simulink model "Battery_Model_1cell_param_"  (R2021b)
settings: Solver=ode3  StartTime=0  StopTime=60000  FixedStep=10  RelTol=1e-3
undefined symbols (not defined in the file or in its folder): Cap, Cell_dev_mean, Cell_dev_sigma, Current_exp_high, n_cells, OCV1, OCV10, OCV2, OCV3, OCV4, OCV5, OCV6, OCV7, OCV8, OCV9, pCl1_High, pCl1_Low, pCl1_Mid, pCl2_High, pCl2_Low, pCl2_Mid, pCl3_High, pCl3_Low, pCl3_Mid, pCs1_High, pCs1_Low, pCs1_Mid, pCs2_High, pCs2_Low, pCs2_Mid, pCs3_High, pCs3_Low, pCs3_Mid, pRl1_High, pRl1_Low, pRl1_Mid, pRl2_High, pRl2_Low, pRl2_Mid, pRl3_High, pRl3_Low, pRl3_Mid, pRs1_High, pRs1_Low, pRs1_Mid, pRs2_High, pRs2_Low, pRs2_Mid, pRs3_High, pRs3_Low, pRs3_Mid, pRse1_High, pRse1_Low, pRse1_Mid, pRse2_High, pRse2_Low, pRse2_Mid, pRse3_High, pRse3_Low, pRse3_Mid ... (+6)
libraries: simulink x2, matrix_library x1
(part 1 of 2)
settings Model: Creator=CWI  LastModifiedBy=osy04
settings SolverCC: AlgebraicLoopSolver=TrustRegion
settings DataIOCC: LimitDataPoints=on  SaveFormat=Array  ReturnWorkspaceOutputs=off
settings OptimizationCC: BlockReduction=off  BooleanDataType=off  LifeSpan=inf
settings DebuggingCC: SaveWithParameterizedLinksMsg=none  UnderspecifiedInitializationDetection=Classic  MergeDetectMultiDrivingBlocksExec=none  SignalResolutionControl=TryResolveAllWithWarning  SFUnexpectedBacktrackingDiag=warning  SFNoUnconditionalDefaultTransitionDiag=warning  SFExecutionAtInitializationDiag=none  SFMachineParentedDataDiag=warning  ArithmeticOperatorsInVariantConditions=warning
settings HardwareCC: ProdBitPerPointer=32  ProdBitPerSizeT=32  ProdBitPerPtrDiffT=32  ProdLargestAtomicFloat=None  ProdIntDivRoundTo=Undefined  ProdEndianess=Unspecified  ProdWordSize=32  ProdHWDeviceType=32-bit Generic  TargetUnknown=on
settings ModelReferenceCC: PropagateSignalLabelsOutOfModel=off
settings SFSimCC: SimUseLocalCustomCode=off  CustomCodeUndefinedFunction=UseInterfaceOnly
settings RTWCC: RTWUseLocalCustomCode=off
settings CodeAppCC: StateflowObjectComments=on
settings GRTTargetCC: TargetLangStandard=C89/C90 (ANSI)
settings ConfigComp: CovMetricSettings=dw  CovSaveCumulativeToWorkspaceVar=on  CovSaveSingleToWorkspaceVar=on  CovExternalEMLEnable=off  CovSFcnEnable=off

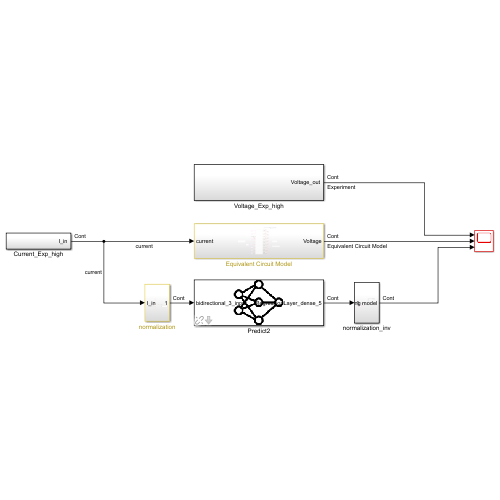
[thumbnail: Simulink's stored preview of the top-level diagram]
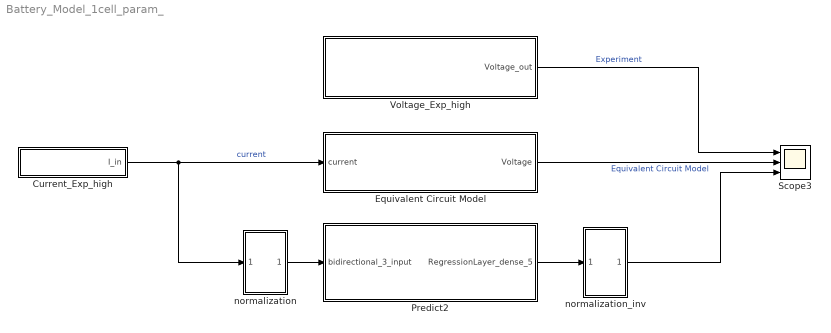
== system Battery_Model_1cell_param_ ==
  Current_Exp_high : Subsystem
  Equivalent Circuit Model : Subsystem
  Predict2 : Subsystem  AncestorBlock=deeplib/Predict  mask(Predict){Network=Network from MAT-file, NetworkFunction=squeezenet, NetworkFilePath=C:\Users\osy04\Desktop\battery_model\Fault detection\code_battery_model_simple\simulink\mymodel_battery_LSTM.mat, MiniBatchSize=32, InputDataFormats={ '', '' }, Predictions=on, Activations={}, ForceInterpretedSim=off, EnableDLNetwork=on}
      mask prompts: Network "deep_blocks:common:Network"; NetworkFunction "deep_blocks:common:MatlabFunction"; NetworkFilePath "deep_blocks:common:FilePath"; MiniBatchSize "deep_blocks:common:MiniBatchSize"; InputDataFormats "deep_blocks:predict:InputDataFormats"; Predictions "deep_blocks:common:Predictions"; Activations "deep_blocks:predict:Activations"; ForceInterpretedSim "deep_blocks:common:ForceInterpretedSim"; EnableDLNetwork "deep_blocks:predict:EnableDlNetwork"
      mask help: deep_blocks:predict:Description
      mask init:
      | deep.blocks.internal.configureDeepNetwork(...
      |     gcb, ...
      |     bdroot, ...
      |     Network, ...
      |     NetworkFilePath, ...
      |     NetworkFunction, ...
      |     MiniBatchSize, ...
      |     logical(Predictions), ...
      |     InputDataFormats, ...
      |     Activations, ...
      |     logical(ForceInterpretedSim), ...
      |     logical(EnableDLNetwork));
      mask Help: helpview('deeplearning', 'nnet_model_predict')
      mask TypeOptions Network: deep_blocks:common:NetworkFromMatFile | deep_blocks:common:NetworkFromFunction | squeezenet
      mask Callback Network:
      | deep.blocks.internal.setNetworkSelectVisibility(gcb);
      | deep.blocks.internal.setDlNetworkOptionsVisibility(gcb);
      | deep.blocks.internal.setActivations(gcb);
      mask Callback NetworkFunction:
      | deep.blocks.internal.setDlNetworkOptionsVisibility(gcb);
      | deep.blocks.internal.setActivations(gcb);
      mask Callback NetworkFilePath:
      | deep.blocks.internal.setDlNetworkOptionsVisibility(gcb);
      | deep.blocks.internal.setActivations(gcb);
      mask TypeOptions Activations: bidirectional_3_input | bidirectional_3 | bidirectional_4 | bidirectional_5 | dense_3 | dense_4 | dense_5
      mask DialogControl Network Prompt: 신경망:
      mask DialogControl NetworkFunction Prompt: MATLAB 함수:
      mask DialogControl NetworkFilePath Prompt: 파일 경로:
      mask DialogControl BrowseButton Prompt: deep_blocks:common:Browse
      mask DialogControl BrowseButton Callback: deep.blocks.internal.handleBrowseButtonClick(gcb);
      mask DialogControl MiniBatchSize Prompt: 미니 배치 크기:
      mask DialogControl InputDataFormats Prompt: 입력 데이터 형식:
      mask DialogControl OutputsContainer Prompt: deep_blocks:common:Outputs
      mask DialogControl Predictions Prompt: 예측
      mask DialogControl ActivationsContainer Prompt: deep_blocks:predict:Activations
      mask DialogControl Activations Prompt: 활성화
      mask DialogControl HiddenContainer Prompt: Hidden Parameters
      mask DialogControl ForceInterpretedSim Prompt: 인터프리터 모드 시뮬레이션 강제 실행
      mask DialogControl EnableDLNetwork Prompt: dlnetwork에 대한 지원 활성화
  Scope3 : Scope  NumInputPorts=3
  Voltage_Exp_high : Subsystem
  normalization : Subsystem
  normalization_inv : Subsystem
  wires:
  normalization/1(Out1) -> Predict2/1(bidirectional_3_input)
  Equivalent Circuit Model/1(Voltage) -> Scope3/2  "Equivalent Circuit Model"
  Voltage_Exp_high/1("Voltage_out ") -> Scope3/1  "Experiment"
  Current_Exp_high/1("I_in ") -> normalization/1("I_in "), Equivalent Circuit Model/1(current)  "current"
  Predict2/1(RegressionLayer_dense_5) -> normalization_inv/1(In1)
  normalization_inv/1(Deep learning model) -> Scope3/3

== system Battery_Model_1cell_param_/Current_Exp_high ==
  Clock : Clock
  "Current " : Constant  Value=Current_exp_high
  Lookup Table Dynamic : simulink/Lookup Tables/Lookup Table Dynamic  LookUpMeth=Interpolation-Use End Values  OutDataType=fixdt('double')  OutScaling=[]  OutputDataTypeScalingMode=Specify via dialog  OutDataTypeStr=fixdt('double')  DoSatur=off
  time : Constant  Value=time_exp_high
  "I_in " : Outport  VectorParamsAs1DForOutWhenUnconnected=off
  wires:
  Lookup Table Dynamic/1 -> "I_in "/1
  Clock/1 -> Lookup Table Dynamic/1
  time/1 -> Lookup Table Dynamic/2
  "Current "/1 -> Lookup Table Dynamic/3

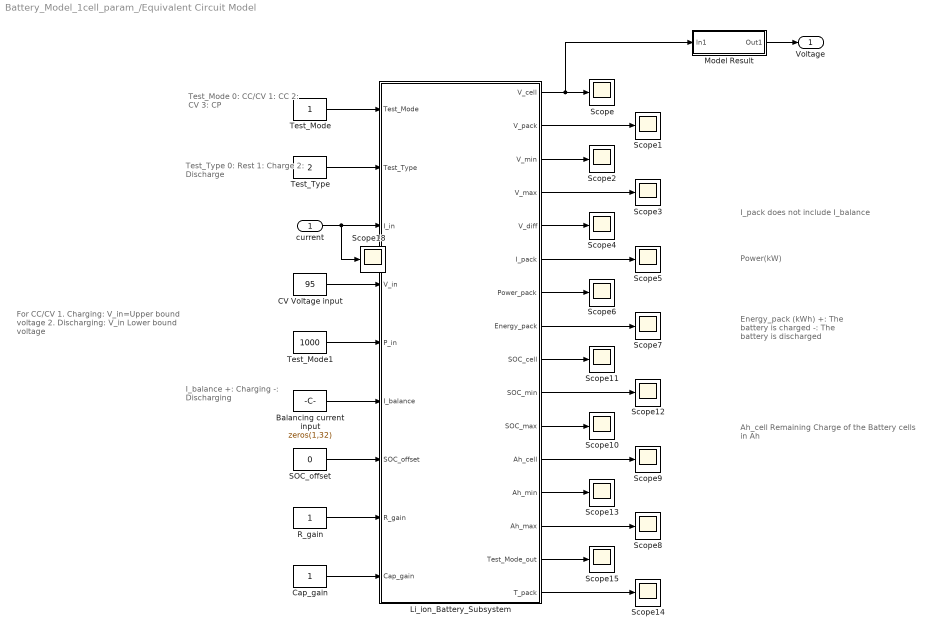
== system Battery_Model_1cell_param_/Equivalent Circuit Model ==
  note: I_balance
      | +: Charging
      | -: Discharging
  note: For CC/CV
      | 1. Charging: V_in=Upper bound voltage
      | 2. Discharging: V_in Lower bound voltage
  note: Test_Mode
      | 0: CC/CV
      | 1: CC
      | 2: CV
      | 3: CP
  note: Test_Type
      | 0: Rest
      | 1: Charge
      | 2: Discharge
  note: I_pack does not include I_balance
  note: Energy_pack (kWh)
      | +: The battery is charged
      | -: The battery is discharged
  note: Ah_cell
      | Remaining Charge of the Battery cells in Ah
  note: Power(kW)
  current : Inport
  Balancing current input : Constant  Value=zeros(1,32)
  CV Voltage input : Constant  Value=95
  Cap_gain : Constant
  Li_ion_Battery_Subsystem : Subsystem
  Model Result : Subsystem
  R_gain : Constant
  SOC_offset : Constant  Value=0
  Scope{,1..15,18} (17 alike) : Scope
  Test_Mode : Constant
  Test_Mode1 : Constant  Value=1000
  Test_Type : Constant  Value=2
  Voltage : Outport  VectorParamsAs1DForOutWhenUnconnected=off
  wires:
  CV Voltage input/1 -> Li_ion_Battery_Subsystem/4(V_in)
  Cap_gain/1 -> Li_ion_Battery_Subsystem/9(Cap_gain)
  Li_ion_Battery_Subsystem/15(Test_Mode_out) -> Scope15/1
  Li_ion_Battery_Subsystem/13(Ah_min) -> Scope13/1
  current/1 -> Scope18/1, Li_ion_Battery_Subsystem/3(I_in)
  Test_Mode/1 -> Li_ion_Battery_Subsystem/1(Test_Mode)
  Li_ion_Battery_Subsystem/14(Ah_max) -> Scope8/1
  Test_Mode1/1 -> Li_ion_Battery_Subsystem/5(P_in)
  Li_ion_Battery_Subsystem/12(Ah_cell) -> Scope9/1
  Li_ion_Battery_Subsystem/16(T_pack) -> Scope14/1
  Test_Type/1 -> Li_ion_Battery_Subsystem/2(Test_Type)
  Li_ion_Battery_Subsystem/8(Energy_pack) -> Scope7/1
  Li_ion_Battery_Subsystem/1(V_cell) -> Model Result/1(In1), Scope/1
  Li_ion_Battery_Subsystem/4(V_max) -> Scope3/1
  Model Result/1(Out1) -> Voltage/1
  Balancing current input/1 -> Li_ion_Battery_Subsystem/6(I_balance)
  Li_ion_Battery_Subsystem/11(SOC_max) -> Scope10/1
  SOC_offset/1 -> Li_ion_Battery_Subsystem/7(SOC_offset)
  R_gain/1 -> Li_ion_Battery_Subsystem/8(R_gain)
  Li_ion_Battery_Subsystem/7(Power_pack) -> Scope6/1
  Li_ion_Battery_Subsystem/3(V_min) -> Scope2/1
  Li_ion_Battery_Subsystem/6(I_pack) -> Scope5/1
  Li_ion_Battery_Subsystem/2(V_pack) -> Scope1/1
  Li_ion_Battery_Subsystem/10(SOC_min) -> Scope12/1
  Li_ion_Battery_Subsystem/9(SOC_cell) -> Scope11/1
  Li_ion_Battery_Subsystem/5(V_diff) -> Scope4/1

== system Battery_Model_1cell_param_/Predict2 ==
  bidirectional_3_input : Inport
  MLFB : MATLAB Function  TreatAsAtomicUnit=on
  RegressionLayer_dense_5 : Outport
  wires:
  bidirectional_3_input/1 -> MLFB/1(in_1)
  MLFB/1(out_1_predict) -> RegressionLayer_dense_5/1

== system Battery_Model_1cell_param_/Voltage_Exp_high ==
  Clock : Clock
  Lookup Table Dynamic : simulink/Lookup Tables/Lookup Table Dynamic  LookUpMeth=Interpolation-Use End Values  OutDataType=fixdt('double')  OutScaling=[]  OutputDataTypeScalingMode=Specify via dialog  OutDataTypeStr=fixdt('double')  DoSatur=off
  time : Constant  Value=time_exp_high
  "voltage " : Constant  Value=Voltage_exp_high
  "Voltage_out " : Outport  VectorParamsAs1DForOutWhenUnconnected=off
  wires:
  Lookup Table Dynamic/1 -> "Voltage_out "/1
  Clock/1 -> Lookup Table Dynamic/1
  time/1 -> Lookup Table Dynamic/2
  "voltage "/1 -> Lookup Table Dynamic/3

== system Battery_Model_1cell_param_/normalization ==
  "I_in " : Inport
  Add : Sum
  Constant : Constant  Value=-0.5
  Display : Display
  Gain : Gain  Gain=1/4
  Mux3 : Mux  Inputs=2
  Reshape : Reshape  OutputDimensionality=Customize  OutputDimensions=[64,2]
  SOC calc : Subsystem
  Scope : Scope
  Scope1 : Scope
  Subsystem1 : Subsystem
  Subsystem4 : Subsystem
  Transpose : matrix_library/Transpose
      settings: SourceProductBaseCode=SL
  oneto64 : Subsystem  Commented=on
  oneto64_2 : Subsystem  Commented=on
  Out1 : Outport
  wires:
  SOC calc/1(Out1) -> Add/1
  "I_in "/1 -> SOC calc/1(In1), Gain/1
  Mux3/1 -> Reshape/1
  Gain/1 -> Subsystem1/1(Inport), Scope1/1
  Add/1 -> Scope/1, Subsystem4/1(Inport)
  Constant/1 -> Add/2
  Reshape/1 -> Transpose/1
  Transpose/1 -> Display/1, Out1/1
  Subsystem4/1(Out1) -> Mux3/2
  Subsystem1/1(Out1) -> Mux3/1

== system Battery_Model_1cell_param_/normalization_inv ==
  In1 : Inport
  Add : Sum
  Constant : Constant  Value=3
  Deep learning model : Outport
  wires:
  Constant/1 -> Add/2
  Add/1 -> Deep learning model/1  "Deep learning model"
  In1/1 -> Add/1

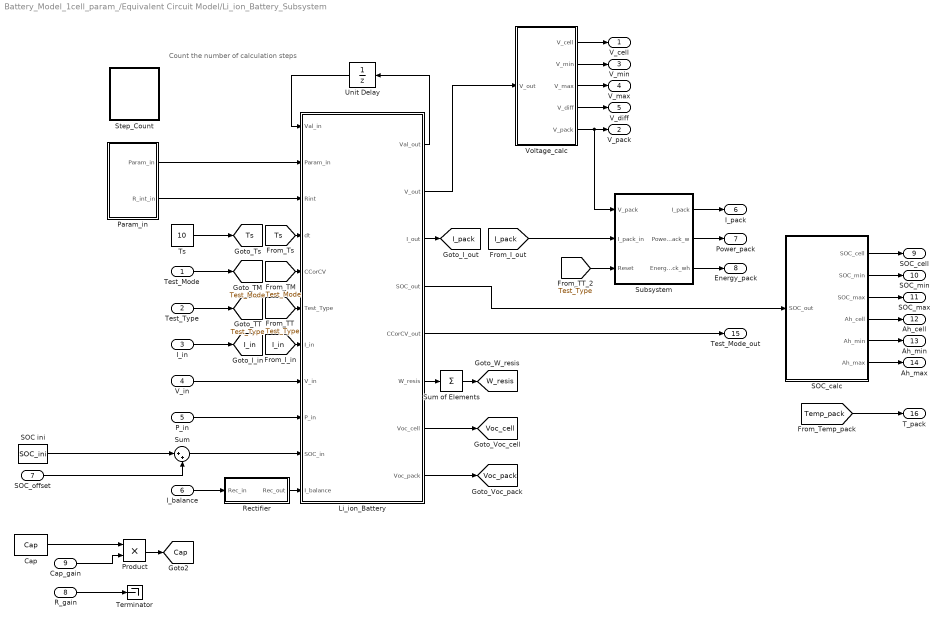
== system Battery_Model_1cell_param_/Equivalent Circuit Model/Li_ion_Battery_Subsystem ==
  note: Count the number of calculation steps
  Test_Mode : Inport
  Test_Type : Inport  Port=2
  I_in : Inport  Port=3
  V_in : Inport  Port=4
  P_in : Inport  Port=5
  I_balance : Inport  Port=6
  SOC_offset : Inport  Port=7
  R_gain : Inport  Port=8
  Cap_gain : Inport  Port=9
  Cap : Constant  Value=Cap
  Li_ion_Battery : MATLAB Function  TreatAsAtomicUnit=on
  Param_in : Subsystem
  Product : Product
  Rectifier : Subsystem
  SOC ini : Constant  Value=SOC_ini
  SOC_calc : Subsystem
  Step_Count : Subsystem
  Subsystem : Subsystem
  Sum : Sum  Inputs=|++
  Sum of Elements : Sum  Inputs=+
  Terminator : Terminator
  Ts : Constant  Value=10
  Unit Delay : UnitDelay  SampleTime=-1  HasFrameUpgradeWarning=on
  Voltage_calc : Subsystem
  V_cell : Outport  VectorParamsAs1DForOutWhenUnconnected=off
  V_pack : Outport  Port=2  VectorParamsAs1DForOutWhenUnconnected=off
  V_min : Outport  Port=3  VectorParamsAs1DForOutWhenUnconnected=off
  V_max : Outport  Port=4  VectorParamsAs1DForOutWhenUnconnected=off
  V_diff : Outport  Port=5  VectorParamsAs1DForOutWhenUnconnected=off
  I_pack : Outport  Port=6  VectorParamsAs1DForOutWhenUnconnected=off
  Power_pack : Outport  Port=7  VectorParamsAs1DForOutWhenUnconnected=off
  Energy_pack : Outport  Port=8  VectorParamsAs1DForOutWhenUnconnected=off
  SOC_cell : Outport  Port=9  VectorParamsAs1DForOutWhenUnconnected=off
  SOC_min : Outport  Port=10  VectorParamsAs1DForOutWhenUnconnected=off
  SOC_max : Outport  Port=11  VectorParamsAs1DForOutWhenUnconnected=off
  Ah_cell : Outport  Port=12  VectorParamsAs1DForOutWhenUnconnected=off
  Ah_min : Outport  Port=13  VectorParamsAs1DForOutWhenUnconnected=off
  Ah_max : Outport  Port=14  VectorParamsAs1DForOutWhenUnconnected=off
  Test_Mode_out : Outport  Port=15  VectorParamsAs1DForOutWhenUnconnected=off
  T_pack : Outport  Port=16  VectorParamsAs1DForOutWhenUnconnected=off
  tag scope: Cap=global, I_in=global, I_pack=global, Test_Mode=global, Test_Type=global, Ts=global, Voc_cell=global, Voc_pack=global, W_resis=global
  wires:
  Param_in/2(R_int_in) -> Li_ion_Battery/3(Rint)
  Unit Delay/1 -> Li_ion_Battery/1(Val_in)
  Li_ion_Battery/1(Val_out) -> Unit Delay/1
  Param_in/1("Param_in ") -> Li_ion_Battery/2(Param_in)
  Li_ion_Battery/5(CCorCV_out) -> Test_Mode_out/1
  Li_ion_Battery/6(W_resis) -> Sum of Elements/1
  Li_ion_Battery/7(Voc_cell) -> [Voc_cell]
  Li_ion_Battery/8(Voc_pack) -> [Voc_pack]
  Li_ion_Battery/3(I_out) -> [I_pack]
  [Temp_pack] -> T_pack/1
  Li_ion_Battery/4(SOC_out) -> SOC_calc/1(SOC_out)
  SOC_calc/2(SOC_min) -> SOC_min/1
  SOC_calc/3(SOC_max) -> SOC_max/1
  SOC_calc/1(SOC_cell) -> SOC_cell/1
  SOC_calc/4(Ah_cell) -> Ah_cell/1
  SOC_calc/5(Ah_min) -> Ah_min/1
  SOC_calc/6(Ah_max) -> Ah_max/1
  Li_ion_Battery/2(V_out) -> Voltage_calc/1(V_out)
  Voltage_calc/2(V_min) -> V_min/1
  Voltage_calc/4(V_diff) -> V_diff/1
  Voltage_calc/3(V_max) -> V_max/1
  Voltage_calc/5(V_pack) -> Subsystem/1(V_pack), V_pack/1
  Voltage_calc/1(V_cell) -> V_cell/1
  [I_pack] -> Subsystem/2(I_pack_in)
  Subsystem/1(I_pack) -> I_pack/1
  Subsystem/2(Power_pack_w) -> Power_pack/1
  Subsystem/3(Energy_pack_wh) -> Energy_pack/1
  Sum of Elements/1 -> [W_resis]
  [Test_Type] -> Subsystem/3(Reset)
  I_balance/1 -> Rectifier/1(Rec_in)
  V_in/1 -> Li_ion_Battery/8(V_in)
  [Ts] -> Li_ion_Battery/4(dt)
  Ts/1 -> [Ts]
  I_in/1 -> [I_in]
  [I_in] -> Li_ion_Battery/7(I_in)
  Rectifier/1(Rec_out) -> Li_ion_Battery/11(I_balance)
  Test_Mode/1 -> [Test_Mode]
  [Test_Mode] -> Li_ion_Battery/5(CCorCV)
  Test_Type/1 -> [Test_Type]
  [Test_Type] -> Li_ion_Battery/6(Test_Type)
  P_in/1 -> Li_ion_Battery/9(P_in)
  Sum/1 -> Li_ion_Battery/10(SOC_in)
  SOC ini/1 -> Sum/1
  SOC_offset/1 -> Sum/2
  Cap/1 -> Product/1
  Product/1 -> [Cap]
  Cap_gain/1 -> Product/2
  R_gain/1 -> Terminator/1

== system Battery_Model_1cell_param_/Equivalent Circuit Model/Model Result ==
  In1 : Inport
  Divide : Product  Inputs=*/
  Sum of Elements : Sum  Inputs=+
  n_cells : Constant  Value=n_cells
  Out1 : Outport  VectorParamsAs1DForOutWhenUnconnected=off
  wires:
  Sum of Elements/1 -> Divide/1
  Divide/1 -> Out1/1
  n_cells/1 -> Divide/2
  In1/1 -> Sum of Elements/1

== system Battery_Model_1cell_param_/normalization/SOC calc ==
  In1 : Inport
  Add : Sum
  Constant : Constant  Value=3600
  Delay4 : Delay  DelayLength=1
  Divide : Product  Inputs=*/
  Gain : Gain  Gain=-1
  Product : Product
  Product1 : Product
  SOC ini : Constant  Value=SOC_ini
  Subtract : Sum  Inputs=+-
  Ts : Constant  Value=10
  Ts1 : Constant  Value=Cap
  Out1 : Outport
  wires:
  Ts/1 -> Product/1
  Ts1/1 -> Product1/1
  SOC ini/1 -> Subtract/1
  Divide/1 -> Gain/1
  Delay4/1 -> Add/2
  Product/1 -> Add/1
  Product1/1 -> Divide/2
  In1/1 -> Product/2
  Add/1 -> Divide/1, Delay4/1
  Constant/1 -> Product1/2
  Subtract/1 -> Out1/1
  Gain/1 -> Subtract/2

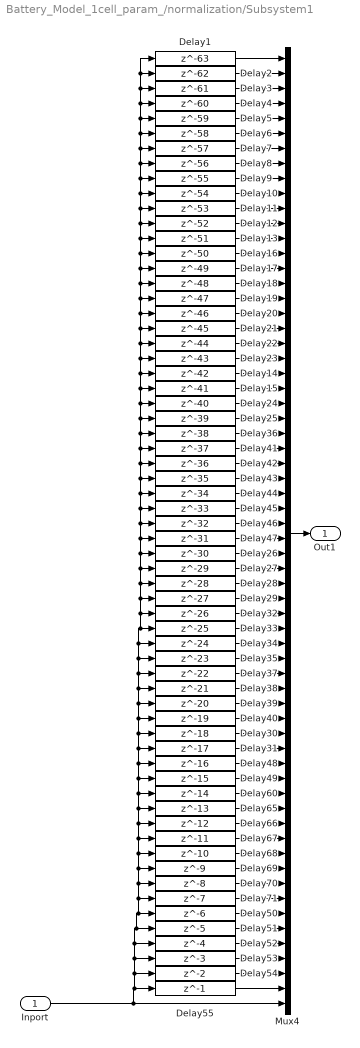
== system Battery_Model_1cell_param_/normalization/Subsystem1 ==
  Inport : Inport
  Delay1 : Delay  DelayLength=63
  Delay10 : Delay  DelayLength=54
  Delay11 : Delay  DelayLength=53
  Delay12 : Delay  DelayLength=52
  Delay13 : Delay  DelayLength=51
  Delay14 : Delay  DelayLength=42
  Delay15 : Delay  DelayLength=41
  Delay16 : Delay  DelayLength=50
  Delay17 : Delay  DelayLength=49
  Delay18 : Delay  DelayLength=48
  Delay19 : Delay  DelayLength=47
  Delay2 : Delay  DelayLength=62
  Delay20 : Delay  DelayLength=46
  Delay21 : Delay  DelayLength=45
  Delay22 : Delay  DelayLength=44
  Delay23 : Delay  DelayLength=43
  Delay24 : Delay  DelayLength=40
  Delay25 : Delay  DelayLength=39
  Delay26 : Delay  DelayLength=30
  Delay27 : Delay  DelayLength=29
  Delay28 : Delay  DelayLength=28
  Delay29 : Delay  DelayLength=27
  Delay3 : Delay  DelayLength=61
  Delay30 : Delay  DelayLength=18
  Delay31 : Delay  DelayLength=17
  Delay32 : Delay  DelayLength=26
  Delay33 : Delay  DelayLength=25
  Delay34 : Delay  DelayLength=24
  Delay35 : Delay  DelayLength=23
  Delay36 : Delay  DelayLength=38
  Delay37 : Delay  DelayLength=22
  Delay38 : Delay  DelayLength=21
  Delay39 : Delay  DelayLength=20
  Delay4 : Delay  DelayLength=60
  Delay40 : Delay  DelayLength=19
  Delay41 : Delay  DelayLength=37
  Delay42 : Delay  DelayLength=36
  Delay43 : Delay  DelayLength=35
  Delay44 : Delay  DelayLength=34
  Delay45 : Delay  DelayLength=33
  Delay46 : Delay  DelayLength=32
  Delay47 : Delay  DelayLength=31
  Delay48 : Delay  DelayLength=16
  Delay49 : Delay  DelayLength=15
  Delay5 : Delay  DelayLength=59
  Delay50 : Delay  DelayLength=6
  Delay51 : Delay  DelayLength=5
  Delay52 : Delay  DelayLength=4
  Delay53 : Delay  DelayLength=3
  Delay54 : Delay
  Delay55 : Delay  DelayLength=1
  Delay6 : Delay  DelayLength=58
  Delay60 : Delay  DelayLength=14
  Delay65 : Delay  DelayLength=13
  Delay66 : Delay  DelayLength=12
  Delay67 : Delay  DelayLength=11
  Delay68 : Delay  DelayLength=10
  Delay69 : Delay  DelayLength=9
  Delay7 : Delay  DelayLength=57
  Delay70 : Delay  DelayLength=8
  Delay71 : Delay  DelayLength=7
  Delay8 : Delay  DelayLength=56
  Delay9 : Delay  DelayLength=55
  Mux4 : Mux  Inputs=64
  Out1 : Outport
  wires:
  Inport/1 -> Mux4/64, Delay55/1, Delay54/1, Delay53/1, Delay52/1, Delay51/1, Delay50/1, Delay71/1, Delay70/1, Delay69/1, Delay68/1, Delay67/1, Delay66/1, Delay65/1, Delay60/1, Delay49/1, Delay48/1, Delay31/1, Delay30/1, Delay40/1, Delay39/1, Delay38/1, Delay37/1, Delay35/1, Delay34/1, Delay33/1, Delay32/1, Delay29/1, Delay28/1, Delay27/1, Delay26/1, Delay47/1, Delay46/1, Delay45/1, Delay44/1, Delay43/1, Delay42/1, Delay41/1, Delay36/1, Delay25/1, Delay24/1, Delay15/1, Delay14/1, Delay23/1, Delay22/1, Delay21/1, Delay20/1, Delay19/1, Delay18/1, Delay17/1, Delay16/1, Delay13/1, Delay12/1, Delay11/1, Delay10/1, Delay9/1, Delay8/1, Delay7/1, Delay6/1, Delay5/1, Delay4/1, Delay3/1, Delay2/1, Delay1/1
  Mux4/1 -> Out1/1
  Delay1/1 -> Mux4/1
  Delay2/1 -> Mux4/2
  Delay3/1 -> Mux4/3
  Delay4/1 -> Mux4/4
  Delay5/1 -> Mux4/5
  Delay6/1 -> Mux4/6
  Delay7/1 -> Mux4/7
  Delay8/1 -> Mux4/8
  Delay9/1 -> Mux4/9
  Delay10/1 -> Mux4/10
  Delay11/1 -> Mux4/11
  Delay12/1 -> Mux4/12
  Delay13/1 -> Mux4/13
  Delay16/1 -> Mux4/14
  Delay17/1 -> Mux4/15
  Delay18/1 -> Mux4/16
  Delay19/1 -> Mux4/17
  Delay20/1 -> Mux4/18
  Delay21/1 -> Mux4/19
  Delay22/1 -> Mux4/20
  Delay23/1 -> Mux4/21
  Delay14/1 -> Mux4/22
  Delay15/1 -> Mux4/23
  Delay24/1 -> Mux4/24
  Delay25/1 -> Mux4/25
  Delay36/1 -> Mux4/26
  Delay41/1 -> Mux4/27
  Delay42/1 -> Mux4/28
  Delay43/1 -> Mux4/29
  Delay44/1 -> Mux4/30
  Delay45/1 -> Mux4/31
  Delay46/1 -> Mux4/32
  Delay47/1 -> Mux4/33
  Delay26/1 -> Mux4/34
  Delay27/1 -> Mux4/35
  Delay28/1 -> Mux4/36
  Delay29/1 -> Mux4/37
  Delay32/1 -> Mux4/38
  Delay33/1 -> Mux4/39
  Delay34/1 -> Mux4/40
  Delay35/1 -> Mux4/41
  Delay37/1 -> Mux4/42
  Delay38/1 -> Mux4/43
  Delay39/1 -> Mux4/44
  Delay40/1 -> Mux4/45
  Delay30/1 -> Mux4/46
  Delay31/1 -> Mux4/47
  Delay48/1 -> Mux4/48
  Delay49/1 -> Mux4/49
  Delay60/1 -> Mux4/50
  Delay65/1 -> Mux4/51
  Delay66/1 -> Mux4/52
  Delay67/1 -> Mux4/53
  Delay68/1 -> Mux4/54
  Delay69/1 -> Mux4/55
  Delay70/1 -> Mux4/56
  Delay71/1 -> Mux4/57
  Delay50/1 -> Mux4/58
  Delay51/1 -> Mux4/59
  Delay52/1 -> Mux4/60
  Delay53/1 -> Mux4/61
  Delay54/1 -> Mux4/62
  Delay55/1 -> Mux4/63

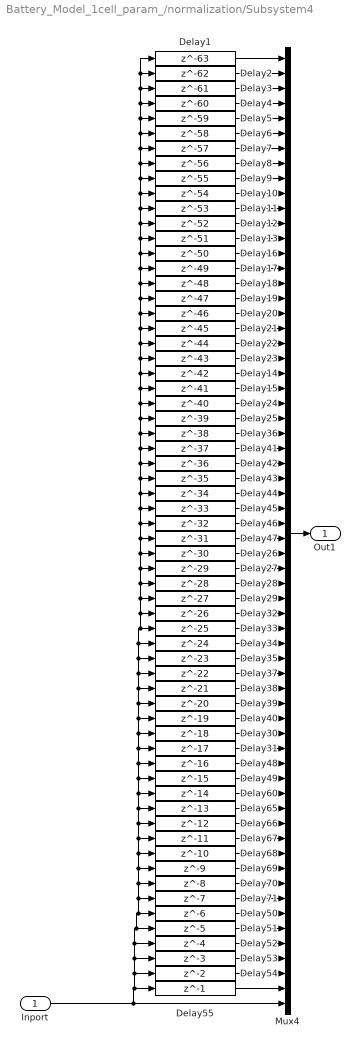
== system Battery_Model_1cell_param_/normalization/Subsystem4 ==
  Inport : Inport
  Delay1 : Delay  DelayLength=63
  Delay10 : Delay  DelayLength=54
  Delay11 : Delay  DelayLength=53
  Delay12 : Delay  DelayLength=52
  Delay13 : Delay  DelayLength=51
  Delay14 : Delay  DelayLength=42
  Delay15 : Delay  DelayLength=41
  Delay16 : Delay  DelayLength=50
  Delay17 : Delay  DelayLength=49
  Delay18 : Delay  DelayLength=48
  Delay19 : Delay  DelayLength=47
  Delay2 : Delay  DelayLength=62
  Delay20 : Delay  DelayLength=46
  Delay21 : Delay  DelayLength=45
  Delay22 : Delay  DelayLength=44
  Delay23 : Delay  DelayLength=43
  Delay24 : Delay  DelayLength=40
  Delay25 : Delay  DelayLength=39
  Delay26 : Delay  DelayLength=30
  Delay27 : Delay  DelayLength=29
  Delay28 : Delay  DelayLength=28
  Delay29 : Delay  DelayLength=27
  Delay3 : Delay  DelayLength=61
  Delay30 : Delay  DelayLength=18
  Delay31 : Delay  DelayLength=17
  Delay32 : Delay  DelayLength=26
  Delay33 : Delay  DelayLength=25
  Delay34 : Delay  DelayLength=24
  Delay35 : Delay  DelayLength=23
  Delay36 : Delay  DelayLength=38
  Delay37 : Delay  DelayLength=22
  Delay38 : Delay  DelayLength=21
  Delay39 : Delay  DelayLength=20
  Delay4 : Delay  DelayLength=60
  Delay40 : Delay  DelayLength=19
  Delay41 : Delay  DelayLength=37
  Delay42 : Delay  DelayLength=36
  Delay43 : Delay  DelayLength=35
  Delay44 : Delay  DelayLength=34
  Delay45 : Delay  DelayLength=33
  Delay46 : Delay  DelayLength=32
  Delay47 : Delay  DelayLength=31
  Delay48 : Delay  DelayLength=16
  Delay49 : Delay  DelayLength=15
  Delay5 : Delay  DelayLength=59
  Delay50 : Delay  DelayLength=6
  Delay51 : Delay  DelayLength=5
  Delay52 : Delay  DelayLength=4
  Delay53 : Delay  DelayLength=3
  Delay54 : Delay
  Delay55 : Delay  DelayLength=1
  Delay6 : Delay  DelayLength=58
  Delay60 : Delay  DelayLength=14
  Delay65 : Delay  DelayLength=13
  Delay66 : Delay  DelayLength=12
  Delay67 : Delay  DelayLength=11
  Delay68 : Delay  DelayLength=10
  Delay69 : Delay  DelayLength=9
  Delay7 : Delay  DelayLength=57
  Delay70 : Delay  DelayLength=8
  Delay71 : Delay  DelayLength=7
  Delay8 : Delay  DelayLength=56
  Delay9 : Delay  DelayLength=55
  Mux4 : Mux  Inputs=64
  Out1 : Outport
  wires:
  Delay55/1 -> Mux4/63
  Delay54/1 -> Mux4/62
  Delay53/1 -> Mux4/61
  Delay52/1 -> Mux4/60
  Delay51/1 -> Mux4/59
  Delay50/1 -> Mux4/58
  Delay71/1 -> Mux4/57
  Delay70/1 -> Mux4/56
  Delay69/1 -> Mux4/55
  Delay68/1 -> Mux4/54
  Delay67/1 -> Mux4/53
  Delay66/1 -> Mux4/52
  Delay65/1 -> Mux4/51
  Delay60/1 -> Mux4/50
  Delay49/1 -> Mux4/49
  Delay48/1 -> Mux4/48
  Delay31/1 -> Mux4/47
  Delay30/1 -> Mux4/46
  Delay40/1 -> Mux4/45
  Delay39/1 -> Mux4/44
  Delay38/1 -> Mux4/43
  Delay37/1 -> Mux4/42
  Delay35/1 -> Mux4/41
  Delay34/1 -> Mux4/40
  Delay33/1 -> Mux4/39
  Delay32/1 -> Mux4/38
  Delay29/1 -> Mux4/37
  Delay28/1 -> Mux4/36
  Delay27/1 -> Mux4/35
  Delay26/1 -> Mux4/34
  Delay47/1 -> Mux4/33
  Delay46/1 -> Mux4/32
  Delay45/1 -> Mux4/31
  Delay44/1 -> Mux4/30
  Delay43/1 -> Mux4/29
  Delay42/1 -> Mux4/28
  Delay41/1 -> Mux4/27
  Delay36/1 -> Mux4/26
  Delay25/1 -> Mux4/25
  Delay24/1 -> Mux4/24
  Delay15/1 -> Mux4/23
  Delay14/1 -> Mux4/22
  Delay23/1 -> Mux4/21
  Delay22/1 -> Mux4/20
  Delay21/1 -> Mux4/19
  Delay20/1 -> Mux4/18
  Delay19/1 -> Mux4/17
  Delay18/1 -> Mux4/16
  Delay17/1 -> Mux4/15
  Delay16/1 -> Mux4/14
  Delay13/1 -> Mux4/13
  Delay12/1 -> Mux4/12
  Delay11/1 -> Mux4/11
  Delay10/1 -> Mux4/10
  Delay9/1 -> Mux4/9
  Delay8/1 -> Mux4/8
  Delay7/1 -> Mux4/7
  Delay6/1 -> Mux4/6
  Delay5/1 -> Mux4/5
  Delay4/1 -> Mux4/4
  Delay3/1 -> Mux4/3
  Delay2/1 -> Mux4/2
  Delay1/1 -> Mux4/1
  Mux4/1 -> Out1/1
  Inport/1 -> Delay1/1, Delay2/1, Delay3/1, Delay4/1, Delay5/1, Delay6/1, Delay7/1, Delay8/1, Delay9/1, Delay10/1, Delay11/1, Delay12/1, Delay13/1, Delay16/1, Delay17/1, Delay18/1, Delay19/1, Delay20/1, Delay21/1, Delay22/1, Delay23/1, Delay14/1, Delay15/1, Delay24/1, Delay25/1, Delay36/1, Delay41/1, Delay42/1, Delay43/1, Delay44/1, Delay45/1, Delay46/1, Delay47/1, Delay26/1, Delay27/1, Delay28/1, Delay29/1, Delay32/1, Delay33/1, Delay34/1, Delay35/1, Delay37/1, Delay38/1, Delay39/1, Delay40/1, Delay30/1, Delay31/1, Delay48/1, Delay49/1, Delay60/1, Delay65/1, Delay66/1, Delay67/1, Delay68/1, Delay69/1, Delay70/1, Delay71/1, Delay50/1, Delay51/1, Delay52/1, Delay53/1, Delay54/1, Delay55/1, Mux4/64

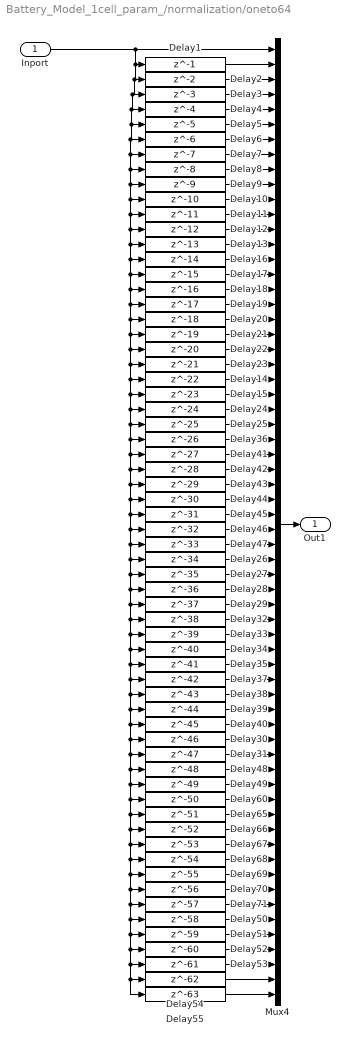
== system Battery_Model_1cell_param_/normalization/oneto64 ==
  Inport : Inport
  Delay1 : Delay  DelayLength=1
  Delay10 : Delay  DelayLength=10
  Delay11 : Delay  DelayLength=11
  Delay12 : Delay  DelayLength=12
  Delay13 : Delay  DelayLength=13
  Delay14 : Delay  DelayLength=22
  Delay15 : Delay  DelayLength=23
  Delay16 : Delay  DelayLength=14
  Delay17 : Delay  DelayLength=15
  Delay18 : Delay  DelayLength=16
  Delay19 : Delay  DelayLength=17
  Delay2 : Delay
  Delay20 : Delay  DelayLength=18
  Delay21 : Delay  DelayLength=19
  Delay22 : Delay  DelayLength=20
  Delay23 : Delay  DelayLength=21
  Delay24 : Delay  DelayLength=24
  Delay25 : Delay  DelayLength=25
  Delay26 : Delay  DelayLength=34
  Delay27 : Delay  DelayLength=35
  Delay28 : Delay  DelayLength=36
  Delay29 : Delay  DelayLength=37
  Delay3 : Delay  DelayLength=3
  Delay30 : Delay  DelayLength=46
  Delay31 : Delay  DelayLength=47
  Delay32 : Delay  DelayLength=38
  Delay33 : Delay  DelayLength=39
  Delay34 : Delay  DelayLength=40
  Delay35 : Delay  DelayLength=41
  Delay36 : Delay  DelayLength=26
  Delay37 : Delay  DelayLength=42
  Delay38 : Delay  DelayLength=43
  Delay39 : Delay  DelayLength=44
  Delay4 : Delay  DelayLength=4
  Delay40 : Delay  DelayLength=45
  Delay41 : Delay  DelayLength=27
  Delay42 : Delay  DelayLength=28
  Delay43 : Delay  DelayLength=29
  Delay44 : Delay  DelayLength=30
  Delay45 : Delay  DelayLength=31
  Delay46 : Delay  DelayLength=32
  Delay47 : Delay  DelayLength=33
  Delay48 : Delay  DelayLength=48
  Delay49 : Delay  DelayLength=49
  Delay5 : Delay  DelayLength=5
  Delay50 : Delay  DelayLength=58
  Delay51 : Delay  DelayLength=59
  Delay52 : Delay  DelayLength=60
  Delay53 : Delay  DelayLength=61
  Delay54 : Delay  DelayLength=62
  Delay55 : Delay  DelayLength=63
  Delay6 : Delay  DelayLength=6
  Delay60 : Delay  DelayLength=50
  Delay65 : Delay  DelayLength=51
  Delay66 : Delay  DelayLength=52
  Delay67 : Delay  DelayLength=53
  Delay68 : Delay  DelayLength=54
  Delay69 : Delay  DelayLength=55
  Delay7 : Delay  DelayLength=7
  Delay70 : Delay  DelayLength=56
  Delay71 : Delay  DelayLength=57
  Delay8 : Delay  DelayLength=8
  Delay9 : Delay  DelayLength=9
  Mux4 : Mux  Inputs=64
  Out1 : Outport
  wires:
  Mux4/1 -> Out1/1
  Delay16/1 -> Mux4/15
  Delay12/1 -> Mux4/13
  Delay11/1 -> Mux4/12
  Delay4/1 -> Mux4/5
  Delay7/1 -> Mux4/8
  Delay6/1 -> Mux4/7
  Delay1/1 -> Mux4/2
  Delay55/1 -> Mux4/64
  Delay52/1 -> Mux4/61
  Delay53/1 -> Mux4/62
  Delay71/1 -> Mux4/58
  Delay51/1 -> Mux4/60
  Delay70/1 -> Mux4/57
  Delay68/1 -> Mux4/55
  Delay30/1 -> Mux4/47
  Delay13/1 -> Mux4/14
  Delay40/1 -> Mux4/46
  Delay49/1 -> Mux4/50
  Delay34/1 -> Mux4/41
  Delay26/1 -> Mux4/35
  Delay37/1 -> Mux4/43
  Delay44/1 -> Mux4/31
  Delay45/1 -> Mux4/32
  Delay46/1 -> Mux4/33
  Delay42/1 -> Mux4/29
  Delay14/1 -> Mux4/23
  Delay27/1 -> Mux4/36
  Delay28/1 -> Mux4/37
  Delay36/1 -> Mux4/27
  Delay15/1 -> Mux4/24
  Delay23/1 -> Mux4/22
  Delay3/1 -> Mux4/4
  Delay41/1 -> Mux4/28
  Delay5/1 -> Mux4/6
  Delay54/1 -> Mux4/63
  Delay8/1 -> Mux4/9
  Delay22/1 -> Mux4/21
  Delay39/1 -> Mux4/45
  Delay10/1 -> Mux4/11
  Delay29/1 -> Mux4/38
  Delay21/1 -> Mux4/20
  Delay32/1 -> Mux4/39
  Delay33/1 -> Mux4/40
  Delay19/1 -> Mux4/18
  Delay9/1 -> Mux4/10
  Delay66/1 -> Mux4/53
  Delay2/1 -> Mux4/3
  Delay60/1 -> Mux4/51
  Delay25/1 -> Mux4/26
  Delay67/1 -> Mux4/54
  Delay48/1 -> Mux4/49
  Delay43/1 -> Mux4/30
  Delay31/1 -> Mux4/48
  Delay35/1 -> Mux4/42
  Delay47/1 -> Mux4/34
  Delay20/1 -> Mux4/19
  Delay18/1 -> Mux4/17
  Inport/1 -> Delay1/1, Delay2/1, Delay3/1, Delay4/1, Delay5/1, Delay6/1, Delay7/1, Delay8/1, Delay9/1, Delay10/1, Delay11/1, Delay12/1, Delay13/1, Delay16/1, Delay17/1, Delay18/1, Delay19/1, Delay20/1, Delay21/1, Delay22/1, Delay23/1, Delay14/1, Delay15/1, Delay24/1, Delay25/1, Delay36/1, Delay41/1, Delay42/1, Delay43/1, Delay44/1, Delay45/1, Delay46/1, Delay47/1, Delay26/1, Delay27/1, Delay28/1, Delay29/1, Delay32/1, Delay33/1, Delay34/1, Delay35/1, Delay37/1, Delay38/1, Delay39/1, Delay40/1, Delay30/1, Delay31/1, Delay48/1, Delay49/1, Delay60/1, Delay65/1, Delay66/1, Delay67/1, Delay68/1, Delay69/1, Delay70/1, Delay71/1, Delay50/1, Delay51/1, Delay52/1, Delay53/1, Delay54/1, Delay55/1, Mux4/1
  Delay69/1 -> Mux4/56
  Delay24/1 -> Mux4/25
  Delay17/1 -> Mux4/16
  Delay65/1 -> Mux4/52
  Delay38/1 -> Mux4/44
  Delay50/1 -> Mux4/59

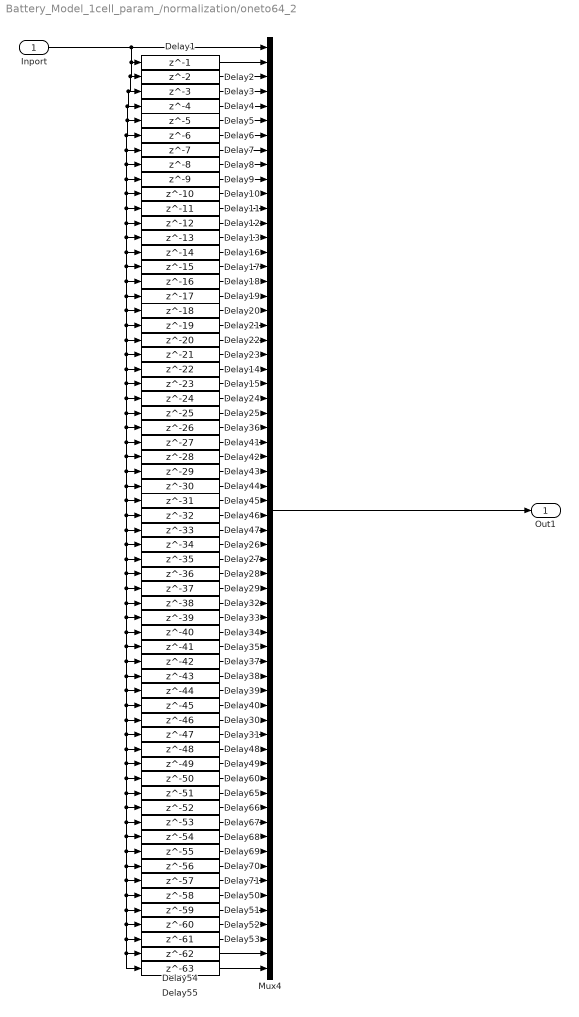
== system Battery_Model_1cell_param_/normalization/oneto64_2 ==
  Inport : Inport
  Delay1 : Delay  DelayLength=1
  Delay10 : Delay  DelayLength=10
  Delay11 : Delay  DelayLength=11
  Delay12 : Delay  DelayLength=12
  Delay13 : Delay  DelayLength=13
  Delay14 : Delay  DelayLength=22
  Delay15 : Delay  DelayLength=23
  Delay16 : Delay  DelayLength=14
  Delay17 : Delay  DelayLength=15
  Delay18 : Delay  DelayLength=16
  Delay19 : Delay  DelayLength=17
  Delay2 : Delay
  Delay20 : Delay  DelayLength=18
  Delay21 : Delay  DelayLength=19
  Delay22 : Delay  DelayLength=20
  Delay23 : Delay  DelayLength=21
  Delay24 : Delay  DelayLength=24
  Delay25 : Delay  DelayLength=25
  Delay26 : Delay  DelayLength=34
  Delay27 : Delay  DelayLength=35
  Delay28 : Delay  DelayLength=36
  Delay29 : Delay  DelayLength=37
  Delay3 : Delay  DelayLength=3
  Delay30 : Delay  DelayLength=46
  Delay31 : Delay  DelayLength=47
  Delay32 : Delay  DelayLength=38
  Delay33 : Delay  DelayLength=39
  Delay34 : Delay  DelayLength=40
  Delay35 : Delay  DelayLength=41
  Delay36 : Delay  DelayLength=26
  Delay37 : Delay  DelayLength=42
  Delay38 : Delay  DelayLength=43
  Delay39 : Delay  DelayLength=44
  Delay4 : Delay  DelayLength=4
  Delay40 : Delay  DelayLength=45
  Delay41 : Delay  DelayLength=27
  Delay42 : Delay  DelayLength=28
  Delay43 : Delay  DelayLength=29
  Delay44 : Delay  DelayLength=30
  Delay45 : Delay  DelayLength=31
  Delay46 : Delay  DelayLength=32
  Delay47 : Delay  DelayLength=33
  Delay48 : Delay  DelayLength=48
  Delay49 : Delay  DelayLength=49
  Delay5 : Delay  DelayLength=5
  Delay50 : Delay  DelayLength=58
  Delay51 : Delay  DelayLength=59
  Delay52 : Delay  DelayLength=60
  Delay53 : Delay  DelayLength=61
  Delay54 : Delay  DelayLength=62
  Delay55 : Delay  DelayLength=63
  Delay6 : Delay  DelayLength=6
  Delay60 : Delay  DelayLength=50
  Delay65 : Delay  DelayLength=51
  Delay66 : Delay  DelayLength=52
  Delay67 : Delay  DelayLength=53
  Delay68 : Delay  DelayLength=54
  Delay69 : Delay  DelayLength=55
  Delay7 : Delay  DelayLength=7
  Delay70 : Delay  DelayLength=56
  Delay71 : Delay  DelayLength=57
  Delay8 : Delay  DelayLength=8
  Delay9 : Delay  DelayLength=9
  Mux4 : Mux  Inputs=64
  Out1 : Outport
  wires:
  Delay50/1 -> Mux4/59
  Delay38/1 -> Mux4/44
  Delay65/1 -> Mux4/52
  Delay17/1 -> Mux4/16
  Delay24/1 -> Mux4/25
  Delay69/1 -> Mux4/56
  Inport/1 -> Mux4/1, Delay55/1, Delay54/1, Delay53/1, Delay52/1, Delay51/1, Delay50/1, Delay71/1, Delay70/1, Delay69/1, Delay68/1, Delay67/1, Delay66/1, Delay65/1, Delay60/1, Delay49/1, Delay48/1, Delay31/1, Delay30/1, Delay40/1, Delay39/1, Delay38/1, Delay37/1, Delay35/1, Delay34/1, Delay33/1, Delay32/1, Delay29/1, Delay28/1, Delay27/1, Delay26/1, Delay47/1, Delay46/1, Delay45/1, Delay44/1, Delay43/1, Delay42/1, Delay41/1, Delay36/1, Delay25/1, Delay24/1, Delay15/1, Delay14/1, Delay23/1, Delay22/1, Delay21/1, Delay20/1, Delay19/1, Delay18/1, Delay17/1, Delay16/1, Delay13/1, Delay12/1, Delay11/1, Delay10/1, Delay9/1, Delay8/1, Delay7/1, Delay6/1, Delay5/1, Delay4/1, Delay3/1, Delay2/1, Delay1/1
  Delay18/1 -> Mux4/17
  Delay20/1 -> Mux4/19
  Delay47/1 -> Mux4/34
  Delay35/1 -> Mux4/42
  Delay31/1 -> Mux4/48
  Delay43/1 -> Mux4/30
  Delay48/1 -> Mux4/49
  Delay67/1 -> Mux4/54
  Delay25/1 -> Mux4/26
  Delay60/1 -> Mux4/51
  Delay2/1 -> Mux4/3
  Delay66/1 -> Mux4/53
  Delay9/1 -> Mux4/10
  Delay19/1 -> Mux4/18
  Delay33/1 -> Mux4/40
  Delay32/1 -> Mux4/39
  Delay21/1 -> Mux4/20
  Delay29/1 -> Mux4/38
  Delay10/1 -> Mux4/11
  Delay39/1 -> Mux4/45
  Delay22/1 -> Mux4/21
  Delay8/1 -> Mux4/9
  Delay54/1 -> Mux4/63
  Delay5/1 -> Mux4/6
  Delay41/1 -> Mux4/28
  Delay3/1 -> Mux4/4
  Delay23/1 -> Mux4/22
  Delay15/1 -> Mux4/24
  Delay36/1 -> Mux4/27
  Delay28/1 -> Mux4/37
  Delay27/1 -> Mux4/36
  Delay14/1 -> Mux4/23
  Delay42/1 -> Mux4/29
  Delay46/1 -> Mux4/33
  Delay45/1 -> Mux4/32
  Delay44/1 -> Mux4/31
  Delay37/1 -> Mux4/43
  Delay26/1 -> Mux4/35
  Delay34/1 -> Mux4/41
  Delay49/1 -> Mux4/50
  Delay40/1 -> Mux4/46
  Delay13/1 -> Mux4/14
  Delay30/1 -> Mux4/47
  Delay68/1 -> Mux4/55
  Delay70/1 -> Mux4/57
  Delay51/1 -> Mux4/60
  Delay71/1 -> Mux4/58
  Delay53/1 -> Mux4/62
  Delay52/1 -> Mux4/61
  Delay55/1 -> Mux4/64
  Delay1/1 -> Mux4/2
  Delay6/1 -> Mux4/7
  Delay7/1 -> Mux4/8
  Delay4/1 -> Mux4/5
  Delay11/1 -> Mux4/12
  Delay12/1 -> Mux4/13
  Delay16/1 -> Mux4/15
  Mux4/1 -> Out1/1

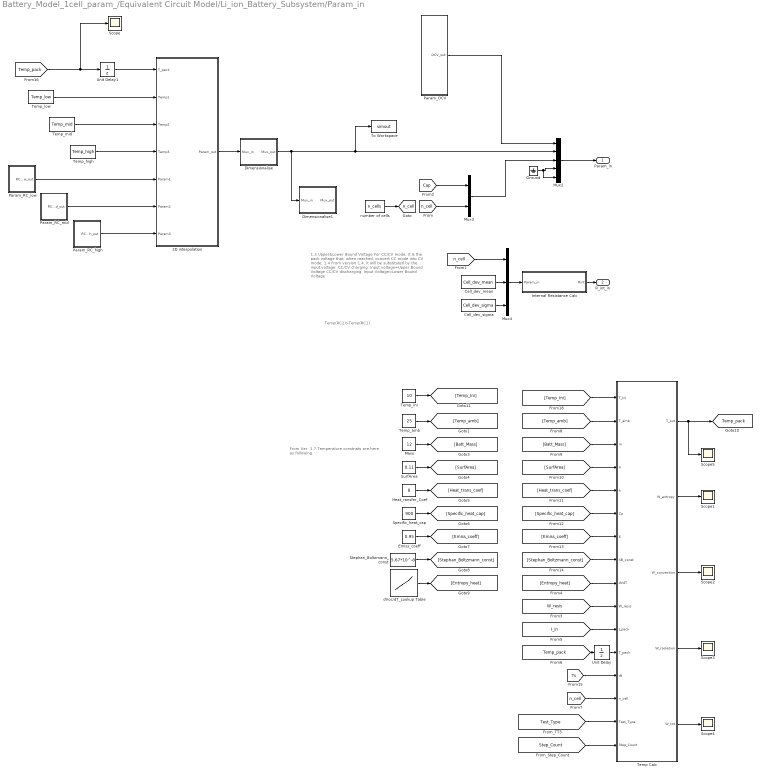
== system Battery_Model_1cell_param_/Equivalent Circuit Model/Li_ion_Battery_Subsystem/Param_in ==
  note: Temp(RC2)>Temp(RC1)
  note: From Ver. 1.7
      | Temperature constnats are here as following
  note: 1.3
      | Upper&Lower Bound Voltage
      | For CC/CV mode, it is the pack voltage
      | that, when reached, convert CC mode
      | into CV mode.
      |
      | 1.4
      | From version 1.4, it will be substituted by
      | the input voltage.
      | CC/CV charging: Input voltage=Upper Bound Voltage
      | CC/CV discharging: Input Voltage=Lower Bound Voltage
  2D interpolation : MATLAB Function  TreatAsAtomicUnit=on
  "Cell_dev_mean " : Constant  Value=Cell_dev_mean
  Cell_dev_sigma : Constant  Value=Cell_dev_sigma
  Dimensionalise : Subsystem
  Dimensionalise1 : Subsystem
  Emiss_coeff : Constant  Value=0.95
  Ground : Ground
  Heat_ransfer_Coef : Constant  Value=8
  Internal Resistance Calc : MATLAB Function  TreatAsAtomicUnit=on
  Mass : Constant  Value=12
  Mux2 : Mux  Inputs=5
  Mux3 : Mux  Inputs=2
  Mux4 : Mux  Inputs=3
  Param_OCV : Subsystem
  Param_RC_high : Subsystem
  Param_RC_low : Subsystem
  Param_RC_mid : Subsystem
  Scope{,1..5} (6 alike) : Scope
  Specific_heat_cap : Constant  Value=900
  Stephan_Boltzmann_const : Constant  Value=5.67*10^-8
  SurfArea : Constant  Value=0.11
  Temp Calc : MATLAB Function  TreatAsAtomicUnit=on
  Temp_Ini : Constant  Value=10
  Temp_amb : Constant  Value=25
  Temp_high : Constant  Value=Temp_high
  Temp_low : Constant  Value=Temp_low
  Temp_mid : Constant  Value=Temp_mid
  To Workspace : ToWorkspace  VariableName=simout  SaveFormat=Timeseries  SampleTime=-1
  Unit Delay : UnitDelay  SampleTime=-1  HasFrameUpgradeWarning=on
  Unit Delay1 : UnitDelay  SampleTime=-1  HasFrameUpgradeWarning=on
  dVoc/dT_Lookup Table : Lookup_n-D  NumberOfTableDimensions=1  BreakpointsForDimension1=[-5:5]  Table=zeros(1,11)  InternalRulePriority=Speed  RndMeth=Simplest  InputSameDT=on
  number of cells : Constant  Value=n_cells
  "Param_in " : Outport  VectorParamsAs1DForOutWhenUnconnected=off
  R_int_in : Outport  Port=2  VectorParamsAs1DForOutWhenUnconnected=off
  tag scope: Temp_pack=global, n_cell=global
  wires:
  Mux4/1 -> Internal Resistance Calc/1(Param_in)
  Mux2/1 -> "Param_in "/1
  Mux3/1 -> Mux2/3
  Cell_dev_sigma/1 -> Mux4/3
  "Cell_dev_mean "/1 -> Mux4/2
  number of cells/1 -> [n_cell]
  [n_cell] -> Mux3/2
  [n_cell] -> Mux4/1
  [Cap] -> Mux3/1
  Temp_amb/1 -> [Temp_amb]
  Mass/1 -> [Batt_Mass]
  SurfArea/1 -> [SurfArea]
  Heat_ransfer_Coef/1 -> [Heat_trans_coef]
  Specific_heat_cap/1 -> [Specific_heat_cap]
  Emiss_coeff/1 -> [Emiss_coeff]
  Stephan_Boltzmann_const/1 -> [Stephan_Boltzmann_const]
  dVoc/dT_Lookup Table/1 -> [Entropy_heat]
  [Temp_amb] -> Temp Calc/2(T_amb)
  [Batt_Mass] -> Temp Calc/3(m)
  [SurfArea] -> Temp Calc/4(A)
  [Heat_trans_coef] -> Temp Calc/5(h)
  [Specific_heat_cap] -> Temp Calc/6(Cp)
  [Emiss_coeff] -> Temp Calc/7(E)
  [Stephan_Boltzmann_const] -> Temp Calc/8(SB_const)
  [Entropy_heat] -> Temp Calc/9(dVdT)
  [W_resis] -> Temp Calc/10(W_resis)
  [I_in] -> Temp Calc/11(I_pack)
  [Ts] -> Temp Calc/13(dt)
  Temp Calc/1(T_out) -> Scope5/1, [Temp_pack]
  Temp Calc/2(W_entropy) -> Scope1/1
  Temp Calc/3(W_convection) -> Scope2/1
  Temp Calc/4(W_radiation) -> Scope3/1
  Temp Calc/5(W_tot) -> Scope4/1
  [Temp_pack] -> Unit Delay/1
  Unit Delay/1 -> Temp Calc/12(T_pack)
  Dimensionalise/1(Mux_out) -> Dimensionalise1/1(Mux_in), To Workspace/1, Mux2/2
  Internal Resistance Calc/1(Rint) -> R_int_in/1
  Param_OCV/1(OCV_out) -> Mux2/1
  [n_cell] -> Temp Calc/14(n_cell)
  [Test_Type] -> Temp Calc/15(Test_Type)
  Temp_Ini/1 -> [Temp_Ini]
  [Temp_Ini] -> Temp Calc/1(T_Ini)
  [Step_Count] -> Temp Calc/16(Step_Count)
  Param_RC_high/1(RC_high_out) -> 2D interpolation/7(Param3)
  Temp_high/1 -> 2D interpolation/4(Temp3)
  Param_RC_mid/1(RC_mid_out) -> 2D interpolation/6(Param2)
  Temp_mid/1 -> 2D interpolation/3(Temp2)
  Param_RC_low/1(RC_low_out) -> 2D interpolation/5(Param1)
  Temp_low/1 -> 2D interpolation/2(Temp1)
  [Temp_pack] -> Scope/1, Unit Delay1/1
  Unit Delay1/1 -> 2D interpolation/1(T_pack)
  2D interpolation/1(Param_out) -> Dimensionalise/1(Mux_in)
  Ground/1 -> Mux2/5, Mux2/4

== system Battery_Model_1cell_param_/Equivalent Circuit Model/Li_ion_Battery_Subsystem/Rectifier ==
  Rec_in : Inport
  MATLAB Function : MATLAB Function  TreatAsAtomicUnit=on
  lo : Constant  Value=-0.005
  up : Constant  Value=0.005
  Rec_out : Outport  VectorParamsAs1DForOutWhenUnconnected=off
  wires:
  up/1 -> MATLAB Function/1(up)
  lo/1 -> MATLAB Function/3(lo)
  Rec_in/1 -> MATLAB Function/2(in)
  MATLAB Function/1(out) -> Rec_out/1

== system Battery_Model_1cell_param_/Equivalent Circuit Model/Li_ion_Battery_Subsystem/SOC_calc ==
  SOC_out : Inport
  Max1 : MinMax  Function=max
  Max2 : MinMax  Function=max
  Min1 : MinMax
  Min2 : MinMax
  Product3 : Product
  SOC_cell : Outport  VectorParamsAs1DForOutWhenUnconnected=off
  SOC_min : Outport  Port=2  VectorParamsAs1DForOutWhenUnconnected=off
  SOC_max : Outport  Port=3  VectorParamsAs1DForOutWhenUnconnected=off
  Ah_cell : Outport  Port=4  VectorParamsAs1DForOutWhenUnconnected=off
  Ah_min : Outport  Port=5  VectorParamsAs1DForOutWhenUnconnected=off
  Ah_max : Outport  Port=6  VectorParamsAs1DForOutWhenUnconnected=off
  wires:
  Min1/1 -> SOC_min/1
  Min2/1 -> Ah_min/1
  SOC_out/1 -> Min1/1, Max1/1, SOC_cell/1, Product3/1
  Max1/1 -> SOC_max/1
  Product3/1 -> Ah_cell/1, Max2/1, Min2/1
  [Cap] -> Product3/2
  Max2/1 -> Ah_max/1

== system Battery_Model_1cell_param_/Equivalent Circuit Model/Li_ion_Battery_Subsystem/Step_Count ==
  note: Initial step에서만 계산되는 값 처리
  Add : Sum
  Constant : Constant
  Delay : Delay  DelayLength=1  InitialCondition=0
  tag scope: Step_Count=global
  wires:
  Delay/1 -> Add/2
  Add/1 -> Delay/1, [Step_Count]
  Constant/1 -> Add/1

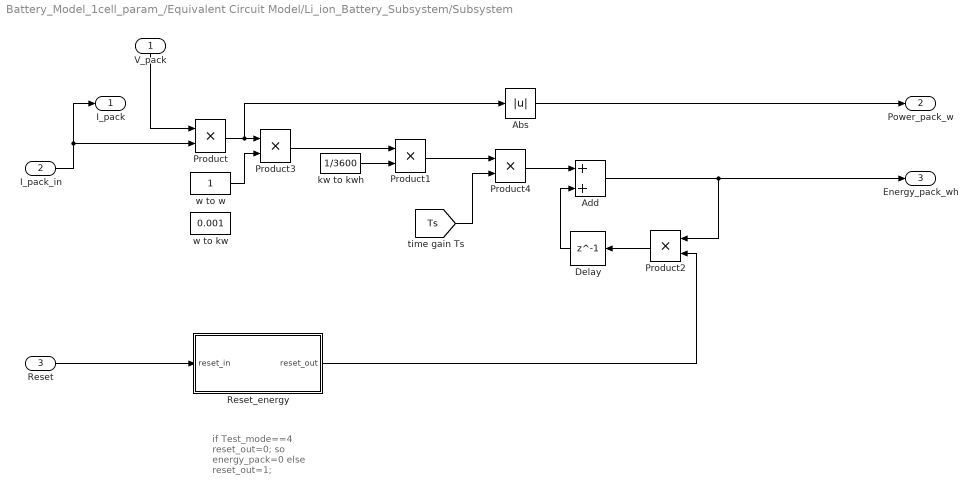
== system Battery_Model_1cell_param_/Equivalent Circuit Model/Li_ion_Battery_Subsystem/Subsystem ==
  note: if Test_mode==4
      | reset_out=0;
      | so energy_pack=0
      | else reset_out=1;
  V_pack : Inport
  I_pack_in : Inport  Port=2
  Reset : Inport  Port=3
  Abs : Abs
  Add : Sum
  Delay : Delay  DelayLength=1  InitialCondition=0
  Product{,1..4} (5 alike) : Product
  Reset_energy : MATLAB Function  TreatAsAtomicUnit=on
  kw to kwh : Constant  Value=1/3600
  w to kw : Constant  Value=0.001
  w to w : Constant
  I_pack : Outport  VectorParamsAs1DForOutWhenUnconnected=off
  Power_pack_w : Outport  Port=2  VectorParamsAs1DForOutWhenUnconnected=off
  Energy_pack_wh : Outport  Port=3  VectorParamsAs1DForOutWhenUnconnected=off
  wires:
  V_pack/1 -> Product/1
  Delay/1 -> Add/2
  Abs/1 -> Power_pack_w/1
  I_pack_in/1 -> I_pack/1, Product/2
  kw to kwh/1 -> Product1/2
  Add/1 -> Product2/1, Energy_pack_wh/1
  Reset/1 -> Reset_energy/1(reset_in)
  Product2/1 -> Delay/1
  Reset_energy/1(reset_out) -> Product2/2
  Product/1 -> Abs/1, Product3/1
  Product3/1 -> Product1/1
  Product4/1 -> Add/1
  Product1/1 -> Product4/1
  [Ts] -> Product4/2
  w to w/1 -> Product3/2

== system Battery_Model_1cell_param_/Equivalent Circuit Model/Li_ion_Battery_Subsystem/Voltage_calc ==
  V_out : Inport
  Max : MinMax  Function=max
  Min : MinMax
  Subtract : Sum  Inputs=-+
  Sum of Elements : Sum  Inputs=+
  V_cell : Outport  VectorParamsAs1DForOutWhenUnconnected=off
  V_min : Outport  Port=2  VectorParamsAs1DForOutWhenUnconnected=off
  V_max : Outport  Port=3  VectorParamsAs1DForOutWhenUnconnected=off
  V_diff : Outport  Port=4  VectorParamsAs1DForOutWhenUnconnected=off
  V_pack : Outport  Port=5  VectorParamsAs1DForOutWhenUnconnected=off
  wires:
  Max/1 -> V_max/1, Subtract/2
  Subtract/1 -> V_diff/1
  V_out/1 -> V_cell/1, Min/1, Max/1, Sum of Elements/1
  Sum of Elements/1 -> V_pack/1
  Min/1 -> V_min/1, Subtract/1

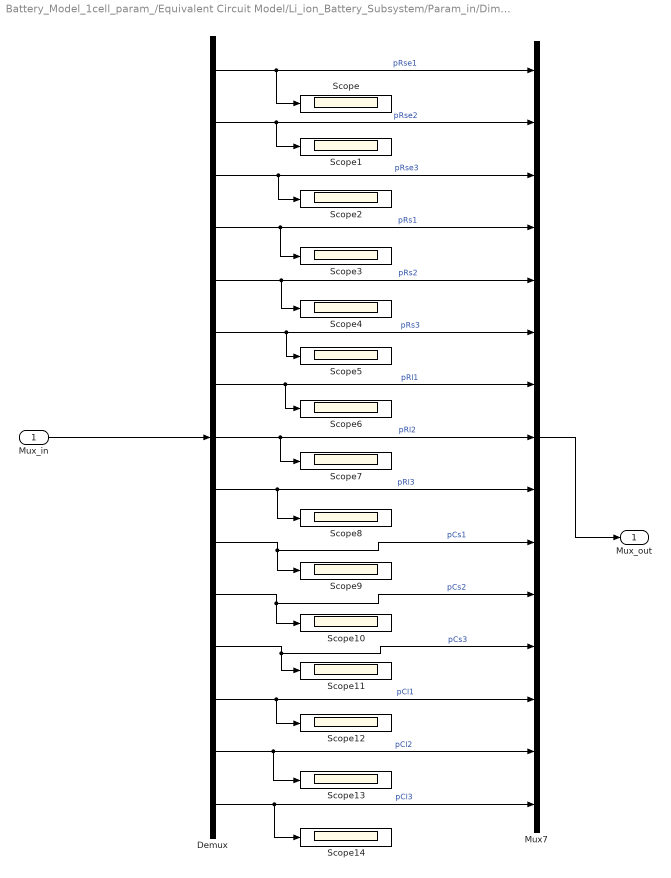
== system Battery_Model_1cell_param_/Equivalent Circuit Model/Li_ion_Battery_Subsystem/Param_in/Dimensionalise ==
  Mux_in : Inport
  Demux : Demux  Outputs=15
  Mux7 : Mux  Inputs=15
  Scope{,1..14} (15 alike) : Scope
  Mux_out : Outport  VectorParamsAs1DForOutWhenUnconnected=off
  wires:
  Mux_in/1 -> Demux/1
  Demux/2 -> Scope1/1, Mux7/2  "pRse2"
  Demux/14 -> Scope13/1, Mux7/14  "pCl2"
  Demux/1 -> Scope/1, Mux7/1  "pRse1"
  Demux/13 -> Scope12/1, Mux7/13  "pCl1"
  Demux/11 -> Scope10/1, Mux7/11  "pCs2"
  Demux/12 -> Scope11/1, Mux7/12  "pCs3"
  Demux/3 -> Scope2/1, Mux7/3  "pRse3"
  Demux/6 -> Scope5/1, Mux7/6  "pRs3"
  Demux/8 -> Scope7/1, Mux7/8  "pRl2"
  Demux/9 -> Scope8/1, Mux7/9  "pRl3"
  Demux/7 -> Scope6/1, Mux7/7  "pRl1"
  Demux/4 -> Scope3/1, Mux7/4  "pRs1"
  Demux/5 -> Scope4/1, Mux7/5  "pRs2"
  Demux/10 -> Scope9/1, Mux7/10  "pCs1"
  Demux/15 -> Scope14/1, Mux7/15  "pCl3"
  Mux7/1 -> Mux_out/1

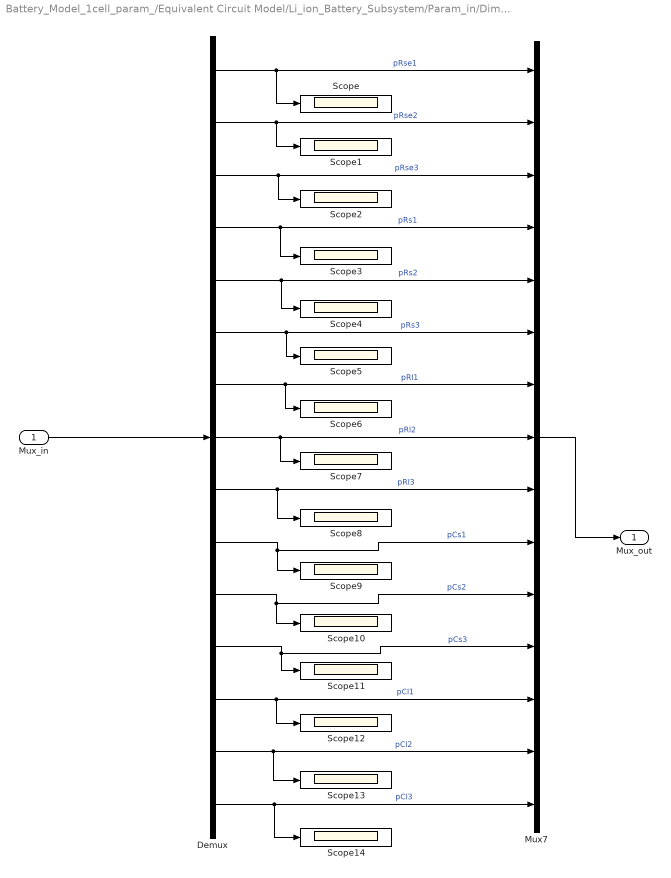
== system Battery_Model_1cell_param_/Equivalent Circuit Model/Li_ion_Battery_Subsystem/Param_in/Dimensionalise1 ==
  Mux_in : Inport
  Demux : Demux  Outputs=15
  Mux7 : Mux  Inputs=15
  Scope{,1..14} (15 alike) : Scope
  Mux_out : Outport  VectorParamsAs1DForOutWhenUnconnected=off
  wires:
  Mux7/1 -> Mux_out/1
  Demux/15 -> Mux7/15, Scope14/1  "pCl3"
  Demux/10 -> Mux7/10, Scope9/1  "pCs1"
  Demux/5 -> Mux7/5, Scope4/1  "pRs2"
  Demux/4 -> Mux7/4, Scope3/1  "pRs1"
  Demux/7 -> Mux7/7, Scope6/1  "pRl1"
  Demux/9 -> Mux7/9, Scope8/1  "pRl3"
  Demux/8 -> Mux7/8, Scope7/1  "pRl2"
  Demux/6 -> Mux7/6, Scope5/1  "pRs3"
  Demux/3 -> Mux7/3, Scope2/1  "pRse3"
  Demux/12 -> Mux7/12, Scope11/1  "pCs3"
  Demux/11 -> Mux7/11, Scope10/1  "pCs2"
  Demux/13 -> Mux7/13, Scope12/1  "pCl1"
  Demux/1 -> Mux7/1, Scope/1  "pRse1"
  Demux/14 -> Mux7/14, Scope13/1  "pCl2"
  Demux/2 -> Mux7/2, Scope1/1  "pRse2"
  Mux_in/1 -> Demux/1

== system Battery_Model_1cell_param_/Equivalent Circuit Model/Li_ion_Battery_Subsystem/Param_in/Param_OCV ==
  Mux1 : Mux  Inputs=10
  OCV1 : Constant  Value=OCV1
  OCV10 : Constant  Value=OCV10
  OCV2 : Constant  Value=OCV2
  OCV3 : Constant  Value=OCV3
  OCV4 : Constant  Value=OCV4
  OCV5 : Constant  Value=OCV5
  OCV6 : Constant  Value=OCV6
  OCV7 : Constant  Value=OCV7
  OCV8 : Constant  Value=OCV8
  OCV9 : Constant  Value=OCV9
  OCV_out : Outport  VectorParamsAs1DForOutWhenUnconnected=off
  wires:
  OCV7/1 -> Mux1/7
  OCV9/1 -> Mux1/9
  OCV10/1 -> Mux1/10
  OCV8/1 -> Mux1/8
  OCV2/1 -> Mux1/2
  OCV5/1 -> Mux1/5
  Mux1/1 -> OCV_out/1
  OCV3/1 -> Mux1/3
  OCV6/1 -> Mux1/6
  OCV4/1 -> Mux1/4
  OCV1/1 -> Mux1/1

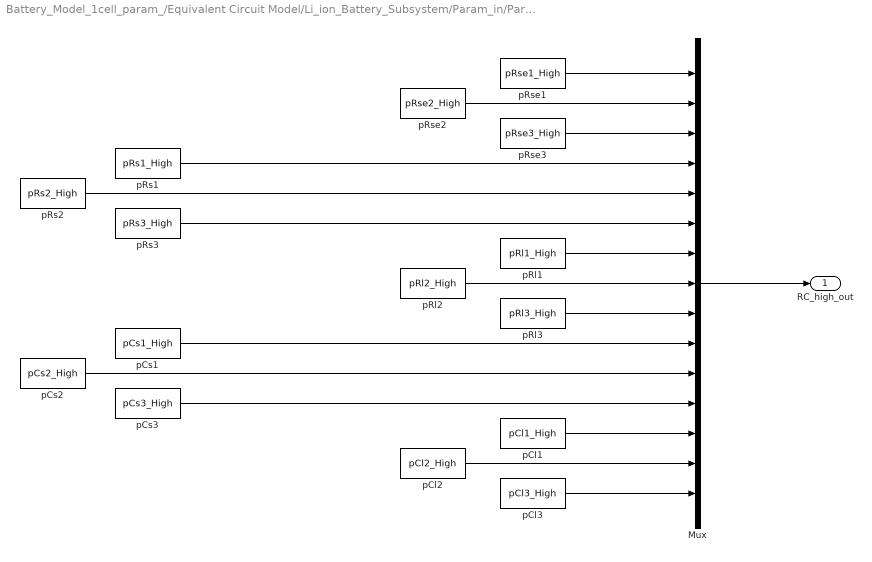
== system Battery_Model_1cell_param_/Equivalent Circuit Model/Li_ion_Battery_Subsystem/Param_in/Param_RC_high ==
  Mux : Mux  Inputs=15
  pCl1 : Constant  Value=pCl1_High
  pCl2 : Constant  Value=pCl2_High
  pCl3 : Constant  Value=pCl3_High
  pCs1 : Constant  Value=pCs1_High
  pCs2 : Constant  Value=pCs2_High
  pCs3 : Constant  Value=pCs3_High
  pRl1 : Constant  Value=pRl1_High
  pRl2 : Constant  Value=pRl2_High
  pRl3 : Constant  Value=pRl3_High
  pRs1 : Constant  Value=pRs1_High
  pRs2 : Constant  Value=pRs2_High
  pRs3 : Constant  Value=pRs3_High
  pRse1 : Constant  Value=pRse1_High
  pRse2 : Constant  Value=pRse2_High
  pRse3 : Constant  Value=pRse3_High
  RC_high_out : Outport  VectorParamsAs1DForOutWhenUnconnected=off
  wires:
  pCs3/1 -> Mux/12
  pRl2/1 -> Mux/8
  pCl2/1 -> Mux/14
  pCs2/1 -> Mux/11
  pRs1/1 -> Mux/4
  Mux/1 -> RC_high_out/1
  pRs3/1 -> Mux/6
  pCl1/1 -> Mux/13
  pCl3/1 -> Mux/15
  pRse2/1 -> Mux/2
  pRl1/1 -> Mux/7
  pRl3/1 -> Mux/9
  pCs1/1 -> Mux/10
  pRs2/1 -> Mux/5
  pRse3/1 -> Mux/3
  pRse1/1 -> Mux/1

== system Battery_Model_1cell_param_/Equivalent Circuit Model/Li_ion_Battery_Subsystem/Param_in/Param_RC_low ==
  Mux : Mux  Inputs=15
  pCl1 : Constant  Value=pCl1_Low
  pCl2 : Constant  Value=pCl2_Low
  pCl3 : Constant  Value=pCl3_Low
  pCs1 : Constant  Value=pCs1_Low
  pCs2 : Constant  Value=pCs2_Low
  pCs3 : Constant  Value=pCs3_Low
  pRl1 : Constant  Value=pRl1_Low
  pRl2 : Constant  Value=pRl2_Low
  pRl3 : Constant  Value=pRl3_Low
  pRs1 : Constant  Value=pRs1_Low
  pRs2 : Constant  Value=pRs2_Low
  pRs3 : Constant  Value=pRs3_Low
  pRse1 : Constant  Value=pRse1_Low
  pRse2 : Constant  Value=pRse2_Low
  pRse3 : Constant  Value=pRse3_Low
  RC_low_out : Outport  VectorParamsAs1DForOutWhenUnconnected=off
  wires:
  pCs3/1 -> Mux/12
  pRl2/1 -> Mux/8
  pCl2/1 -> Mux/14
  pCs2/1 -> Mux/11
  pRs1/1 -> Mux/4
  Mux/1 -> RC_low_out/1
  pRs3/1 -> Mux/6
  pCl1/1 -> Mux/13
  pCl3/1 -> Mux/15
  pRse2/1 -> Mux/2
  pRl1/1 -> Mux/7
  pRl3/1 -> Mux/9
  pCs1/1 -> Mux/10
  pRs2/1 -> Mux/5
  pRse3/1 -> Mux/3
  pRse1/1 -> Mux/1

== system Battery_Model_1cell_param_/Equivalent Circuit Model/Li_ion_Battery_Subsystem/Param_in/Param_RC_mid ==
  Mux : Mux  Inputs=15
  pCl1 : Constant  Value=pCl1_Mid
  pCl2 : Constant  Value=pCl2_Mid
  pCl3 : Constant  Value=pCl3_Mid
  pCs1 : Constant  Value=pCs1_Mid
  pCs2 : Constant  Value=pCs2_Mid
  pCs3 : Constant  Value=pCs3_Mid
  pRl1 : Constant  Value=pRl1_Mid
  pRl2 : Constant  Value=pRl2_Mid
  pRl3 : Constant  Value=pRl3_Mid
  pRs1 : Constant  Value=pRs1_Mid
  pRs2 : Constant  Value=pRs2_Mid
  pRs3 : Constant  Value=pRs3_Mid
  pRse1 : Constant  Value=pRse1_Mid
  pRse2 : Constant  Value=pRse2_Mid
  pRse3 : Constant  Value=pRse3_Mid
  RC_mid_out : Outport  VectorParamsAs1DForOutWhenUnconnected=off
  wires:
  pCs3/1 -> Mux/12
  pRl2/1 -> Mux/8
  pCl2/1 -> Mux/14
  pCs2/1 -> Mux/11
  pRs1/1 -> Mux/4
  Mux/1 -> RC_mid_out/1
  pRs3/1 -> Mux/6
  pCl1/1 -> Mux/13
  pCl3/1 -> Mux/15
  pRse2/1 -> Mux/2
  pRl1/1 -> Mux/7
  pRl3/1 -> Mux/9
  pCs1/1 -> Mux/10
  pRs2/1 -> Mux/5
  pRse3/1 -> Mux/3
  pRse1/1 -> Mux/1

== matlab function Battery_Model_1cell_param_/Equivalent Circuit Model/Li_ion_Battery_Subsystem/Rectifier/MATLAB Function ==
  data: up input; out output; in input; lo input
function out = fcn(up, in, lo)
%#codegen
n_max=32;
out=zeros(1,n_max);
for i=1:n_max
    if (in(i)<up && in(i)>lo)
        out(i)=0;
    else
        out(i)=in(i);
    end
end

== matlab function Battery_Model_1cell_param_/Equivalent Circuit Model/Li_ion_Battery_Subsystem/Subsystem/Reset_energy ==
  data: reset_in input; reset_out output
function reset_out = fcn(reset_in)
%#codegen
% if reset in=4, reset the energy spent to 0

if reset_in==4 
    reset_out=0;
else
    reset_out=1;
end

== matlab function Battery_Model_1cell_param_/Predict2/MLFB ==
  data: in_1 input; out_1_predict output
function out_1_predict  = deepNetwork( in_1 )
[out_1_predict] = deep.blocks.internal.deepNetwork({in_1}, {size(in_1)}, {class(in_1)}, coder.const("Battery_Model_1cell_param_/Predict2"), 'C:\Users\osy04\Desktop\battery_model\Fault detection\code_battery_model_simple\simulink\mymodel_battery_LSTM.mat', false, false, 32, true, {''}, {});
end
